simulink model "Basic_DMT"  (R2014b)
settings: Solver=FixedStepDiscrete  SolverMode=SingleTasking  StartTime=0.0  StopTime=25e-6-14e-9*24  RelTol=1e-3
PreLoadFcn:
  | userName = getenv('UserName');
  | 
  | if strcmp(userName,'Tim')
  | cd C:\Users\Tim\Documents\GitHub\MA_1\Basic_DMT
  | else
  | cd C:\Users\Tim-UML\Documents\GitHub\MA_1\Basic_DMT
  | end
InitFcn:
  | userName = getenv('UserName');
  | 
  | if strcmp(userName,'Tim')
  | cd C:\Users\Tim\Documents\GitHub\MA_1\Basic_DMT
  | else
  | cd C:\Users\Tim-UML\Documents\GitHub\MA_1\Basic_DMT
  | end
values from neighbouring files (symbols this model uses):
  a0 = 0.21194908595403703    (= 0.211949085954)    [initScript.m]
  a1 = 0.576101828091926    (= 0.576101828092)    [initScript.m]
  a2 = a0    (= 0.211949085954)    [initScript.m]
  beta = 1    [initScript.m]
  bitPerSymb = 4    [initScript.m]
  chanDownFact = Tchan/SystemPeriod    [initScript.m]
  fftLen = 16    [initScript.m]
  fftLenActive = fftLenDMT    (= 32)    [initScript.m]
  fftLenDMT = 2*fftLen    (= 32)    [initScript.m]
  GI_Active = GI_LenDMT    (= 0)    [initScript.m]
  GI_Len = 0    [initScript.m]
  GI_LenDMT = 0    [initScript.m]
  M = log2(fftLen)    [initScript.m]
  sysgenSystemPeriod = 4e-9    (= 4e-09)    [initScript.m]
  SystemPeriod = 4e-9    (= 4e-09)    [initScript.m]
  upsampleFactor = 1    [initScript.m]
  usedSubCar = 14    [initScript.m]
undefined symbols (not defined in the file or in its folder): bitCount, get, modu_mode, Tb, Ts
libraries: xbsIndex_r4 x822, commdigbbndam3 x59, simulink x42, dspsigops x7, commrandsrc2 x6, dspbuff3 x4, dspxfrm3 x3, dspswit3 x2, commseqgen2 x1, dsparch4 x1, commutil2 x1, dspsnks4 x1
(part 9 of 10)

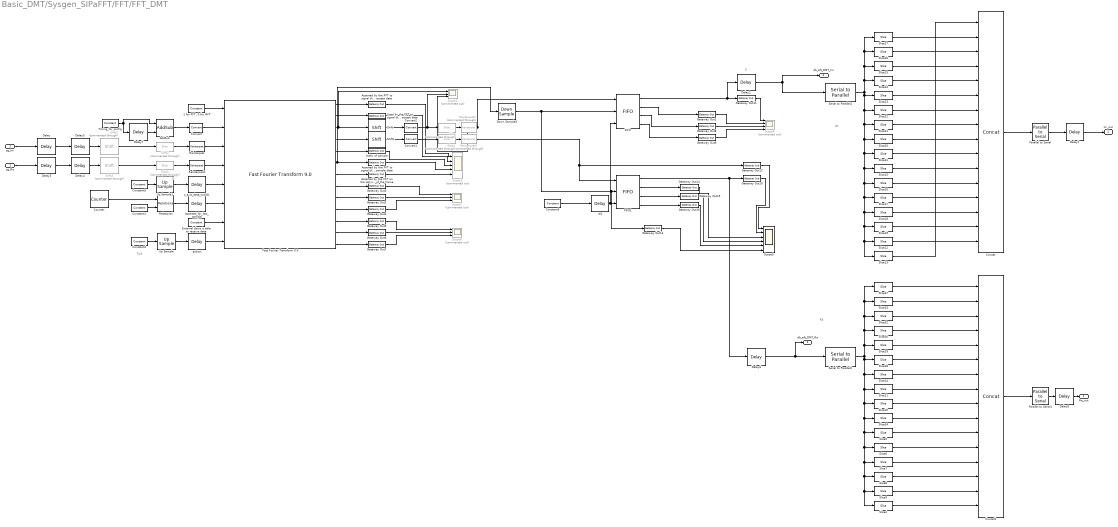
== system Basic_DMT/Sysgen_SIPaFFT/FFT/FFT_DMT ==
  note: 5
  note: IM
  note: RE
  note: 6
  note: Ts/3
  sg_Re : Inport
  sg_Im : Inport  Port=2
  "1 for FFT, 0 for IFFT " : xbsIndex_r4/Constant  const=1  gui_display_data_type=Fixed-point  arith_type=Unsigned  n_bits=1  bin_pt=0  preci_type=Single  exp_width=8  frac_width=24  explicit_period=on  period=Ts  equ=P=C  opselect=C  inp2=PCIN>>17  opr=+  inp1=P  carry=CIN  dbl_ovrd=off  block_type=constant
  AddSub : xbsIndex_r4/AddSub  mode=Subtraction  use_carryin=off  use_carryout=off  en=off  latency=0  precision=User Defined  arith_type=Unsigned  n_bits=1  bin_pt=0  quantization=Truncate  overflow=Wrap  use_behavioral_HDL=off  hw_selection=Fabric  pipelined=off  dbl_ovrd=off  block_type=addsub
  "Asserted by the FFT on the last sample of the frame " : xbsIndex_r4/Gateway Out  inherit_from_input=off  hdl_port=off  rows=1  columns=1  UseAsDAC=off  DACChannel='1'  interface=None  automatic_assignment=on  address_offset=hex2dec('00')  intf_description=''  timing_constraint=None  locs_specified=off  LOCs={}  io_standard={}  block_type=gatewayout
  "Asserted by the FFT to signal that it is ready to accept data " : xbsIndex_r4/Gateway Out  inherit_from_input=off  hdl_port=off  rows=1  columns=1  UseAsDAC=off  DACChannel='1'  interface=None  automatic_assignment=on  address_offset=hex2dec('00')  intf_description=''  timing_constraint=None  locs_specified=off  LOCs={}  io_standard={}  block_type=gatewayout
  Asserted by the FFT to signal that it is ready to provide sample data : xbsIndex_r4/Gateway Out  inherit_from_input=off  hdl_port=off  rows=1  columns=1  UseAsDAC=off  DACChannel='1'  interface=None  automatic_assignment=on  address_offset=hex2dec('00')  intf_description=''  timing_constraint=None  locs_specified=off  LOCs={}  io_standard={}  block_type=gatewayout
  Asserted_for_last_sample : xbsIndex_r4/Delay  rst=off  infoeditControl=Selection of Reset will increase slice count due to use of real FFs and instead of SRLs  en=off  latency=1  reg_retiming=off  dbl_ovrd=off  block_type=delay
  Concat : xbsIndex_r4/Concat  num_inputs=16  dbl_ovrd=off  block_type=concat
  Concat1 : xbsIndex_r4/Concat  num_inputs=16  dbl_ovrd=off  block_type=concat
  Constant1 : xbsIndex_r4/Constant  const=fftLenDMT-1  gui_display_data_type=Fixed-point  arith_type=Unsigned  n_bits=log2(fftLenDMT)  bin_pt=0  preci_type=Single  exp_width=8  frac_width=24  explicit_period=on  period=Ts*usedSubCar*bitPerSymb/fftLenDMT  equ=P=C  opselect=C  inp2=PCIN>>17  opr=+  inp1=P  carry=CIN  dbl_ovrd=off  block_type=constant
  Constant3 : xbsIndex_r4/Constant  const=1  gui_display_data_type=Boolean  arith_type=Boolean  n_bits=1  bin_pt=0  preci_type=Single  exp_width=8  frac_width=24  explicit_period=on  period=Ts*usedSubCar*bitPerSymb/fftLenDMT  equ=P=C  opselect=C  inp2=PCIN>>17  opr=+  inp1=P  carry=CIN  dbl_ovrd=off  block_type=constant
  Constant4 : xbsIndex_r4/Constant  const=1  gui_display_data_type=Boolean  arith_type=Boolean  n_bits=1  bin_pt=0  preci_type=Single  exp_width=8  frac_width=24  explicit_period=on  period=sysgenSystemPeriod*2  equ=P=C  opselect=C  inp2=PCIN>>17  opr=+  inp1=P  carry=CIN  dbl_ovrd=off  block_type=constant
  Constant5 : xbsIndex_r4/Constant  const=1  gui_display_data_type=Boolean  arith_type=Boolean  n_bits=1  bin_pt=0  preci_type=Single  exp_width=8  frac_width=24  explicit_period=on  period=Ts*usedSubCar*bitPerSymb/fftLenDMT  equ=P=C  opselect=C  inp2=PCIN>>17  opr=+  inp1=P  carry=CIN  dbl_ovrd=off  block_type=constant
  Convert : xbsIndex_r4/Convert  gui_display_data_type=Boolean  arith_type=Boolean  n_bits=1  bin_pt=0  float_type=Single  exp_bits=8  fraction_bits=24  quantization=Truncate  overflow=Wrap  en=off  latency=1  pipeline=off  dbl_ovrd=off  block_type=convert
  Convert1 : xbsIndex_r4/Convert  gui_display_data_type=Fixed-point  arith_type="Signed  (2's comp)"  n_bits=bitCount+(log2(fftLen)+1)*2  bin_pt=fracLen  float_type=Single  exp_bits=8  fraction_bits=24  quantization="Round  (unbiased: +/- Inf)"  overflow=Saturate  en=off  latency=0  pipeline=off  dbl_ovrd=off  block_type=convert
  Convert2 : xbsIndex_r4/Convert  gui_display_data_type=Fixed-point  arith_type="Signed  (2's comp)"  n_bits=bitCount+(log2(fftLen)+1)*2  bin_pt=fracLen  float_type=Single  exp_bits=8  fraction_bits=24  quantization="Round  (unbiased: +/- Inf)"  overflow=Saturate  en=off  latency=0  pipeline=off  dbl_ovrd=off  block_type=convert
  Counter : xbsIndex_r4/Counter  cnt_type=Count Limited  cnt_to=fftLenDMT-1  operation=Up  start_count=0  cnt_by_val=1  arith_type=Unsigned  n_bits=log2(fftLenDMT)  bin_pt=0  load_pin=off  rst=off  en=off  explicit_period=on  period=Ts*usedSubCar*bitPerSymb/fftLenDMT  use_behavioral_HDL=off  implementation=Fabric  dbl_ovrd=off  block_type=counter
  Delay : xbsIndex_r4/Delay  rst=off  infoeditControl=Selection of Reset will increase slice count due to use of real FFs and instead of SRLs  en=off  latency=1  reg_retiming=off  dbl_ovrd=off  block_type=delay
  Delay1 : xbsIndex_r4/Delay  rst=off  infoeditControl=Selection of Reset will increase slice count due to use of real FFs and instead of SRLs  en=off  latency=3  reg_retiming=off  dbl_ovrd=off  block_type=delay
  Delay2 : xbsIndex_r4/Delay  rst=off  infoeditControl=Selection of Reset will increase slice count due to use of real FFs and instead of SRLs  en=off  latency=6  reg_retiming=off  dbl_ovrd=off  block_type=delay
  Delay3 : xbsIndex_r4/Delay  rst=off  infoeditControl=Selection of Reset will increase slice count due to use of real FFs and instead of SRLs  en=off  latency=1  reg_retiming=off  dbl_ovrd=off  block_type=delay
  Delay4 : xbsIndex_r4/Delay  rst=off  infoeditControl=Selection of Reset will increase slice count due to use of real FFs and instead of SRLs  en=off  latency=16  reg_retiming=off  dbl_ovrd=off  block_type=delay
  Delay5 : xbsIndex_r4/Delay  rst=off  infoeditControl=Selection of Reset will increase slice count due to use of real FFs and instead of SRLs  en=off  latency=16  reg_retiming=off  dbl_ovrd=off  block_type=delay
  Delay6 : xbsIndex_r4/Delay  rst=off  infoeditControl=Selection of Reset will increase slice count due to use of real FFs and instead of SRLs  en=off  latency=6  reg_retiming=off  dbl_ovrd=off  block_type=delay
  Delay7 : xbsIndex_r4/Delay  rst=off  infoeditControl=Selection of Reset will increase slice count due to use of real FFs and instead of SRLs  en=off  latency=1  reg_retiming=off  dbl_ovrd=off  block_type=delay
  Delay8 : xbsIndex_r4/Delay  rst=off  infoeditControl=Selection of Reset will increase slice count due to use of real FFs and instead of SRLs  en=off  latency=3  reg_retiming=off  dbl_ovrd=off  block_type=delay
  Down Sample5 : xbsIndex_r4/Down Sample  sample_ratio=2  sample_phase=First Value of Frame  en=off  rst=off  latency=0  dbl_ovrd=off  block_type=dsamp
  "Externel slave is able to receive data " : xbsIndex_r4/Constant  const=1  gui_display_data_type=Boolean  arith_type=Boolean  n_bits=1  bin_pt=0  preci_type=Single  exp_width=8  frac_width=24  explicit_period=on  period=Ts  equ=P=C  opselect=C  inp2=PCIN>>17  opr=+  inp1=P  carry=CIN  dbl_ovrd=off  block_type=constant
  FIFO : xbsIndex_r4/FIFO  mem_type=Block RAM  performance_options=Standard_FIFO  embedded_registers=off  depth=32  percent_nbits=4  rst=off  rst_latency=1  en=off  use_dcount=off  use_percent_full_port=on  use_almost_empty=off  almost_empty_thresh=2  use_almost_full=off  almost_full_thresh=14  explicit_period=off  dbl_ovrd=off  block_type=fifo
  FIFO1 : xbsIndex_r4/FIFO  mem_type=Block RAM  performance_options=Standard_FIFO  embedded_registers=off  depth=32  percent_nbits=4  rst=off  rst_latency=1  en=off  use_dcount=off  use_percent_full_port=on  use_almost_empty=off  almost_empty_thresh=2  use_almost_full=off  almost_full_thresh=14  explicit_period=off  dbl_ovrd=off  block_type=fifo
  "Fast Fourier Transform 9.0 " : xbsIndex_r4/Fast Fourier Transform 9.0   transform_length=32  target_clock_frequency=250  target_data_throughput=50  implementation_options=pipelined_streaming_io  run_time_configurable_transform_length=off  phase_factor_width=20  scaling_options=unscaled  rounding_modes=convergent_rounding  aclken=on  aresetn=off  cyclic_prefix_insertion=off  output_ordering=natural_order  throttle_scheme=nonrealtime  xk_index=on  ovflo=off  trim_axipin_name=off  memory_options_data=block_ram  memory_options_phase_factors=block_ram  number_of_stages_using_block_ram_for_data_and_phase_factors=0  memory_options_reorder=block_ram  memory_options_hybrid=off  complex_mult_type=use_mults_resources  butterfly_type=use_xtremedsp_slices  channels=1  input_ordering=natural_order  input_width=16  ip_name=Fast Fourier Transform  ip_version=9.0  dsptool_ready=true  ipcore_usecache=true  ipcore_useipmodelcache=true  wrapper_available=true  port_translation_map={ 'aclken' => 'en', 'aresetn' => 'rst'}  data_format=fixed_point  block_type=xfft_v9_0
  Gateway Out{1..16} (16 alike) : xbsIndex_r4/Gateway Out  inherit_from_input=off  hdl_port=off  rows=1  columns=1  UseAsDAC=off  DACChannel='1'  interface=None  automatic_assignment=on  address_offset=hex2dec('00')  intf_description=''  timing_constraint=None  locs_specified=off  LOCs={}  io_standard={}  block_type=gatewayout
  Index of sample : xbsIndex_r4/Gateway Out  inherit_from_input=off  hdl_port=off  rows=1  columns=1  UseAsDAC=off  DACChannel='1'  interface=None  automatic_assignment=on  address_offset=hex2dec('00')  intf_description=''  timing_constraint=None  locs_specified=off  LOCs={}  io_standard={}  block_type=gatewayout
  Parallel to Serial : xbsIndex_r4/Parallel to Serial  output_order=Most Significant Word First  arith_type=Unsigned  output_bits=(bitCount+(log2(fftLen)+1)*2)  bin_pt=0  rst=off  en=off  latency=1  dbl_ovrd=off  block_type=p2s
      settings: infoedit=Each sample presented at the input becomes several samples presented serially at the output.
  Parallel to Serial1 : xbsIndex_r4/Parallel to Serial  output_order=Most Significant Word First  arith_type=Unsigned  output_bits=(bitCount+(log2(fftLen)+1)*2)  bin_pt=0  rst=off  en=off  latency=1  dbl_ovrd=off  block_type=p2s
      settings: infoedit=Each sample presented at the input becomes several samples presented serially at the output.
  Reinterpret : xbsIndex_r4/Reinterpret  force_arith_type=on  arith_type="Signed  (2's comp)"  force_bin_pt=on  bin_pt=bitCount-1+log2(fftLen)+1  block_type=reinterpret
  Reinterpret1 : xbsIndex_r4/Reinterpret  force_arith_type=on  arith_type="Signed  (2's comp)"  force_bin_pt=on  bin_pt=bitCount-1+log2(fftLen)+1  block_type=reinterpret
  Reinterpret2 : xbsIndex_r4/Reinterpret  Commented=through  force_arith_type=on  arith_type="Signed  (2's comp)"  force_bin_pt=on  bin_pt=fracLen  block_type=reinterpret
  Reinterpret3 : xbsIndex_r4/Reinterpret  Commented=through  force_arith_type=on  arith_type="Signed  (2's comp)"  force_bin_pt=on  bin_pt=fracLen  block_type=reinterpret
  Relational : xbsIndex_r4/Relational  mode=a=b  op_type=Bool  en=off  latency=0  dbl_ovrd=off  block_type=relational
  Scope1 : Scope  Commented=on  NumInputPorts=3
      settings: YMin=-5~-5~-5  YMax=5~5~5  SaveName=ScopeData42
  Scope2 : Scope  Commented=on  NumInputPorts=3
      settings: YMin=-5~-5~-5  YMax=5~5~5  SaveName=ScopeData49
  Scope3 : Scope  Commented=on  NumInputPorts=5
      settings: YMin=-5~-5~-5~-5~-5  YMax=5~5~5~5~5  SaveName=ScopeData51
  Scope4 : Scope  Commented=on  NumInputPorts=4
      settings: YMin=-5~-5~-5~-5  YMax=5~5~5~5  SaveName=ScopeData55
  Scope5 : Scope  NumInputPorts=6
      settings: YMin=-5~-5~-5~-5~-5~-5  YMax=5~5~5~5~5~5  SaveName=ScopeData56
  Scope8 : Scope  Commented=on  NumInputPorts=3
      settings: YMin=-5~-5~-5  YMax=5~5~5  SaveName=ScopeData57
  Serial to Parallel1 : xbsIndex_r4/Serial to Parallel  input_order=Most Significant Word First  arith_type=Unsigned  output_bits=(bitCount+(log2(fftLen)+1)*2)*fftLenDMT  bin_pt=0  rst=off  en=off  latency=1  dbl_ovrd=off  block_type=s2p
      settings: infoedit=Groups of samples presented serially at the input become single samples presented at the output.
  Serial to Parallel2 : xbsIndex_r4/Serial to Parallel  input_order=Most Significant Word First  arith_type=Unsigned  output_bits=(bitCount+(log2(fftLen)+1)*2)*fftLenDMT  bin_pt=0  rst=off  en=off  latency=1  dbl_ovrd=off  block_type=s2p
      settings: infoedit=Groups of samples presented serially at the input become single samples presented at the output.
  Shift : xbsIndex_r4/Shift  shift_dir=Left  shift_bits=2  en=off  latency=0  precision=Full  arith_type="Signed  (2's comp)"  n_bits=13  bin_pt=4  quantization="Round  (unbiased: +/- Inf)"  overflow=Saturate  dbl_ovrd=off  block_type=shift
  Shift1 : xbsIndex_r4/Shift  shift_dir=Left  shift_bits=2  en=off  latency=0  precision=Full  arith_type="Signed  (2's comp)"  n_bits=13  bin_pt=4  quantization="Round  (unbiased: +/- Inf)"  overflow=Saturate  dbl_ovrd=off  block_type=shift
  Shift2 : xbsIndex_r4/Shift  Commented=through  shift_dir=Right  shift_bits=1  en=off  latency=1  precision=Full  arith_type="Signed  (2's comp)"  n_bits=13  bin_pt=4  quantization="Round  (unbiased: +/- Inf)"  overflow=Saturate  dbl_ovrd=off  block_type=shift
  Shift3 : xbsIndex_r4/Shift  Commented=through  shift_dir=Right  shift_bits=1  en=off  latency=1  precision=Full  arith_type="Signed  (2's comp)"  n_bits=13  bin_pt=4  quantization="Round  (unbiased: +/- Inf)"  overflow=Saturate  dbl_ovrd=off  block_type=shift
  Slice : xbsIndex_r4/Slice  Commented=through  nbits=13  boolean_output=off  mode=Lower Bit Location + Width  bit1=0  base1=MSB of Input  bit0=0  base0=LSB of Input  dbl_ovrd=off  block_type=slice
  Slice1 : xbsIndex_r4/Slice  Commented=through  nbits=13  boolean_output=off  mode=Lower Bit Location + Width  bit1=0  base1=MSB of Input  bit0=0  base0=LSB of Input  dbl_ovrd=off  block_type=slice
  Slice10 : xbsIndex_r4/Slice  nbits=(bitCount+(log2(fftLen)+1)*2)  boolean_output=off  mode=Lower Bit Location + Width  bit1=0  base1=LSB of Input  bit0=(bitCount+(log2(fftLen)+1)*2)*23  base0=LSB of Input  dbl_ovrd=off  block_type=slice
  Slice11 : xbsIndex_r4/Slice  nbits=(bitCount+(log2(fftLen)+1)*2)  boolean_output=off  mode=Lower Bit Location + Width  bit1=0  base1=LSB of Input  bit0=(bitCount+(log2(fftLen)+1)*2)*24  base0=LSB of Input  dbl_ovrd=off  block_type=slice
  Slice12 : xbsIndex_r4/Slice  nbits=(bitCount+(log2(fftLen)+1)*2)  boolean_output=off  mode=Lower Bit Location + Width  bit1=0  base1=MSB of Input  bit0=(bitCount+(log2(fftLen)+1)*2)*16  base0=LSB of Input  dbl_ovrd=off  block_type=slice
  Slice13 : xbsIndex_r4/Slice  nbits=(bitCount+(log2(fftLen)+1)*2)  boolean_output=off  mode=Lower Bit Location + Width  bit1=0  base1=MSB of Input  bit0=(bitCount+(log2(fftLen)+1)*2)*15  base0=LSB of Input  dbl_ovrd=off  block_type=slice
  Slice14 : xbsIndex_r4/Slice  nbits=(bitCount+(log2(fftLen)+1)*2)  boolean_output=off  mode=Lower Bit Location + Width  bit1=0  base1=LSB of Input  bit0=(bitCount+(log2(fftLen)+1)*2)*25  base0=LSB of Input  dbl_ovrd=off  block_type=slice
  Slice15 : xbsIndex_r4/Slice  nbits=(bitCount+(log2(fftLen)+1)*2)  boolean_output=off  mode=Lower Bit Location + Width  bit1=24  base1=LSB of Input  bit0=(bitCount+(log2(fftLen)+1)*2)*21  base0=LSB of Input  dbl_ovrd=off  block_type=slice
  Slice16 : xbsIndex_r4/Slice  nbits=(bitCount+(log2(fftLen)+1)*2)  boolean_output=off  mode=Lower Bit Location + Width  bit1=0  base1=MSB of Input  bit0=(bitCount+(log2(fftLen)+1)*2)*20  base0=LSB of Input  dbl_ovrd=off  block_type=slice
  Slice17 : xbsIndex_r4/Slice  nbits=(bitCount+(log2(fftLen)+1)*2)  boolean_output=off  mode=Lower Bit Location + Width  bit1=0  base1=MSB of Input  bit0=(bitCount+(log2(fftLen)+1)*2)*19  base0=LSB of Input  dbl_ovrd=off  block_type=slice
  Slice18 : xbsIndex_r4/Slice  nbits=(bitCount+(log2(fftLen)+1)*2)  boolean_output=off  mode=Lower Bit Location + Width  bit1=0  base1=MSB of Input  bit0=(bitCount+(log2(fftLen)+1)*2)*18  base0=LSB of Input  dbl_ovrd=off  block_type=slice
  Slice19 : xbsIndex_r4/Slice  nbits=(bitCount+(log2(fftLen)+1)*2)  boolean_output=off  mode=Lower Bit Location + Width  bit1=0  base1=MSB of Input  bit0=(bitCount+(log2(fftLen)+1)*2)*17  base0=LSB of Input  dbl_ovrd=off  block_type=slice
  Slice2 : xbsIndex_r4/Slice  Commented=through  nbits=16  boolean_output=off  mode=Lower Bit Location + Width  bit1=0  base1=MSB of Input  bit0=0  base0=LSB of Input  dbl_ovrd=off  block_type=slice
  Slice20 : xbsIndex_r4/Slice  nbits=(bitCount+(log2(fftLen)+1)*2)  boolean_output=off  mode=Lower Bit Location + Width  bit1=0  base1=LSB of Input  bit0=(bitCount+(log2(fftLen)+1)*2)*23  base0=LSB of Input  dbl_ovrd=off  block_type=slice
  Slice21 : xbsIndex_r4/Slice  nbits=(bitCount+(log2(fftLen)+1)*2)  boolean_output=off  mode=Lower Bit Location + Width  bit1=0  base1=LSB of Input  bit0=(bitCount+(log2(fftLen)+1)*2)*24  base0=LSB of Input  dbl_ovrd=off  block_type=slice
  Slice22 : xbsIndex_r4/Slice  nbits=(bitCount+(log2(fftLen)+1)*2)  boolean_output=off  mode=Lower Bit Location + Width  bit1=0  base1=LSB of Input  bit0=(bitCount+(log2(fftLen)+1)*2)*25  base0=LSB of Input  dbl_ovrd=off  block_type=slice
  Slice23 : xbsIndex_r4/Slice  nbits=(bitCount+(log2(fftLen)+1)*2)  boolean_output=off  mode=Lower Bit Location + Width  bit1=0  base1=LSB of Input  bit0=(bitCount+(log2(fftLen)+1)*2)*26  base0=LSB of Input  dbl_ovrd=off  block_type=slice
  Slice24 : xbsIndex_r4/Slice  nbits=(bitCount+(log2(fftLen)+1)*2)  boolean_output=off  mode=Lower Bit Location + Width  bit1=0  base1=LSB of Input  bit0=(bitCount+(log2(fftLen)+1)*2)*27  base0=LSB of Input  dbl_ovrd=off  block_type=slice
  Slice25 : xbsIndex_r4/Slice  nbits=(bitCount+(log2(fftLen)+1)*2)  boolean_output=off  mode=Lower Bit Location + Width  bit1=0  base1=LSB of Input  bit0=(bitCount+(log2(fftLen)+1)*2)*28  base0=LSB of Input  dbl_ovrd=off  block_type=slice
  Slice26 : xbsIndex_r4/Slice  nbits=(bitCount+(log2(fftLen)+1)*2)  boolean_output=off  mode=Lower Bit Location + Width  bit1=0  base1=LSB of Input  bit0=(bitCount+(log2(fftLen)+1)*2)*29  base0=LSB of Input  dbl_ovrd=off  block_type=slice
  Slice27 : xbsIndex_r4/Slice  nbits=(bitCount+(log2(fftLen)+1)*2)  boolean_output=off  mode=Lower Bit Location + Width  bit1=0  base1=LSB of Input  bit0=(bitCount+(log2(fftLen)+1)*2)*30  base0=LSB of Input  dbl_ovrd=off  block_type=slice
  Slice28 : xbsIndex_r4/Slice  nbits=(bitCount+(log2(fftLen)+1)*2)  boolean_output=off  mode=Lower Bit Location + Width  bit1=0  base1=LSB of Input  bit0=(bitCount+(log2(fftLen)+1)*2)*26  base0=LSB of Input  dbl_ovrd=off  block_type=slice
  Slice29 : xbsIndex_r4/Slice  nbits=(bitCount+(log2(fftLen)+1)*2)  boolean_output=off  mode=Lower Bit Location + Width  bit1=0  base1=LSB of Input  bit0=(bitCount+(log2(fftLen)+1)*2)*27  base0=LSB of Input  dbl_ovrd=off  block_type=slice
  Slice3 : xbsIndex_r4/Slice  Commented=through  nbits=16  boolean_output=off  mode=Lower Bit Location + Width  bit1=0  base1=MSB of Input  bit0=0  base0=LSB of Input  dbl_ovrd=off  block_type=slice
  Slice30 : xbsIndex_r4/Slice  nbits=(bitCount+(log2(fftLen)+1)*2)  boolean_output=off  mode=Lower Bit Location + Width  bit1=0  base1=LSB of Input  bit0=(bitCount+(log2(fftLen)+1)*2)*28  base0=LSB of Input  dbl_ovrd=off  block_type=slice
  Slice31 : xbsIndex_r4/Slice  nbits=(bitCount+(log2(fftLen)+1)*2)  boolean_output=off  mode=Lower Bit Location + Width  bit1=0  base1=LSB of Input  bit0=(bitCount+(log2(fftLen)+1)*2)*22  base0=LSB of Input  dbl_ovrd=off  block_type=slice
  Slice32 : xbsIndex_r4/Slice  nbits=(bitCount+(log2(fftLen)+1)*2)  boolean_output=off  mode=Lower Bit Location + Width  bit1=0  base1=LSB of Input  bit0=(bitCount+(log2(fftLen)+1)*2)*29  base0=LSB of Input  dbl_ovrd=off  block_type=slice
  Slice33 : xbsIndex_r4/Slice  nbits=(bitCount+(log2(fftLen)+1)*2)  boolean_output=off  mode=Lower Bit Location + Width  bit1=0  base1=LSB of Input  bit0=(bitCount+(log2(fftLen)+1)*2)*30  base0=LSB of Input  dbl_ovrd=off  block_type=slice
  Slice34 : xbsIndex_r4/Slice  nbits=(bitCount+(log2(fftLen)+1)*2)  boolean_output=off  mode=Lower Bit Location + Width  bit1=0  base1=LSB of Input  bit0=(bitCount+(log2(fftLen)+1)*2)*22  base0=LSB of Input  dbl_ovrd=off  block_type=slice
  Slice37 : xbsIndex_r4/Slice  nbits=(bitCount+(log2(fftLen)+1)*2)  boolean_output=off  mode=Lower Bit Location + Width  bit1=0  base1=LSB of Input  bit0=(bitCount+(log2(fftLen)+1)*2)*31  base0=LSB of Input  dbl_ovrd=off  block_type=slice
  Slice4 : xbsIndex_r4/Slice  nbits=(bitCount+(log2(fftLen)+1)*2)  boolean_output=off  mode=Lower Bit Location + Width  bit1=0  base1=MSB of Input  bit0=(bitCount+(log2(fftLen)+1)*2)*16  base0=LSB of Input  dbl_ovrd=off  block_type=slice
  Slice5 : xbsIndex_r4/Slice  nbits=(bitCount+(log2(fftLen)+1)*2)  boolean_output=off  mode=Lower Bit Location + Width  bit1=24  base1=LSB of Input  bit0=(bitCount+(log2(fftLen)+1)*2)*21  base0=LSB of Input  dbl_ovrd=off  block_type=slice
  Slice6 : xbsIndex_r4/Slice  nbits=(bitCount+(log2(fftLen)+1)*2)  boolean_output=off  mode=Lower Bit Location + Width  bit1=0  base1=MSB of Input  bit0=(bitCount+(log2(fftLen)+1)*2)*20  base0=LSB of Input  dbl_ovrd=off  block_type=slice
  Slice7 : xbsIndex_r4/Slice  nbits=(bitCount+(log2(fftLen)+1)*2)  boolean_output=off  mode=Lower Bit Location + Width  bit1=0  base1=MSB of Input  bit0=(bitCount+(log2(fftLen)+1)*2)*19  base0=LSB of Input  dbl_ovrd=off  block_type=slice
  Slice8 : xbsIndex_r4/Slice  nbits=(bitCount+(log2(fftLen)+1)*2)  boolean_output=off  mode=Lower Bit Location + Width  bit1=0  base1=MSB of Input  bit0=(bitCount+(log2(fftLen)+1)*2)*18  base0=LSB of Input  dbl_ovrd=off  block_type=slice
  Slice9 : xbsIndex_r4/Slice  nbits=(bitCount+(log2(fftLen)+1)*2)  boolean_output=off  mode=Lower Bit Location + Width  bit1=0  base1=MSB of Input  bit0=(bitCount+(log2(fftLen)+1)*2)*17  base0=LSB of Input  dbl_ovrd=off  block_type=slice
  Timing_for_config : xbsIndex_r4/Constant  const=1  gui_display_data_type=Fixed-point  arith_type=Unsigned  n_bits=1  bin_pt=0  preci_type=Single  exp_width=8  frac_width=24  explicit_period=on  period=Ts  equ=P=C  opselect=C  inp2=PCIN>>17  opr=+  inp1=P  carry=CIN  dbl_ovrd=off  block_type=constant
  Up Sample : xbsIndex_r4/Up Sample  sample_ratio=2  copy_samples=off  en=off  latency=0  dbl_ovrd=off  block_type=usamp
  Up Sample1 : xbsIndex_r4/Up Sample  sample_ratio=Ts*usedSubCar*bitPerSymb/fftLenDMT/sysgenSystemPeriod  copy_samples=off  en=off  latency=0  dbl_ovrd=off  block_type=usamp
  Used by the FFT to signal that it is ready to accept data : xbsIndex_r4/Gateway Out  inherit_from_input=off  hdl_port=off  rows=1  columns=1  UseAsDAC=off  DACChannel='1'  interface=None  automatic_assignment=on  address_offset=hex2dec('00')  intf_description=''  timing_constraint=None  locs_specified=off  LOCs={}  io_standard={}  block_type=gatewayout
  "aclken " : xbsIndex_r4/Delay  rst=off  infoeditControl=Selection of Reset will increase slice count due to use of real FFs and instead of SRLs  en=off  latency=1  reg_retiming=off  dbl_ovrd=off  block_type=delay
  re2 : xbsIndex_r4/Delay  rst=off  infoeditControl=Selection of Reset will increase slice count due to use of real FFs and instead of SRLs  en=off  latency=1  reg_retiming=off  dbl_ovrd=off  block_type=delay
  s_axis_data_tvalid1 : xbsIndex_r4/Delay  rst=off  infoeditControl=Selection of Reset will increase slice count due to use of real FFs and instead of SRLs  en=off  latency=1  reg_retiming=off  dbl_ovrd=off  block_type=delay
  Re_out : Outport
  Im_out : Outport  Port=2
  db_aft_DMT_Re : Outport  Port=3
  db_aft_DMT_Im : Outport  Port=4
  wires:
  "1 for FFT, 0 for IFFT "/1 -> "Fast Fourier Transform 9.0 "/1
  "Externel slave is able to receive data "/1 -> "Fast Fourier Transform 9.0 "/7
  "Fast Fourier Transform 9.0 "/4 -> Shift1/1
  Shift1/1 -> Convert1/1
  Slice/1 -> Reinterpret2/1
  Slice1/1 -> Reinterpret3/1
  Slice2/1 -> Reinterpret/1
  Slice3/1 -> Reinterpret1/1
  Shift/1 -> Convert2/1
  Delay/1 -> Delay5/1
  Delay3/1 -> Delay4/1
  Reinterpret2/1 -> FIFO/1, Scope1/3
  Reinterpret1/1 -> "Fast Fourier Transform 9.0 "/4
  Reinterpret/1 -> "Fast Fourier Transform 9.0 "/3
  Shift2/1 -> Slice2/1
  Shift3/1 -> Slice3/1
  Convert2/1 -> Slice/1, Scope1/2
  Convert1/1 -> Slice1/1
  "Fast Fourier Transform 9.0 "/6 -> Asserted by the FFT to signal that it is ready to provide sample data/1, Down Sample5/1
  "Fast Fourier Transform 9.0 "/7 -> "Asserted by the FFT on the last sample of the frame "/1
  "Fast Fourier Transform 9.0 "/10 -> Gateway Out4/1
  "Fast Fourier Transform 9.0 "/11 -> Gateway Out5/1
  "Fast Fourier Transform 9.0 "/12 -> Gateway Out6/1
  "Fast Fourier Transform 9.0 "/13 -> Gateway Out7/1
  "Fast Fourier Transform 9.0 "/9 -> Gateway Out2/1
  "Fast Fourier Transform 9.0 "/8 -> Gateway Out3/1
  Gateway Out6/1 -> Scope8/2
  Gateway Out7/1 -> Scope8/3
  Gateway Out5/1 -> Scope8/1
  Gateway Out2/1 -> Scope2/2
  Gateway Out3/1 -> Scope2/1
  Gateway Out4/1 -> Scope2/3
  Asserted by the FFT to signal that it is ready to provide sample data/1 -> Scope3/4
  "Asserted by the FFT on the last sample of the frame "/1 -> Scope3/5
  Index of sample/1 -> Scope3/3
  Used by the FFT to signal that it is ready to accept data/1 -> Scope3/2
  "Fast Fourier Transform 9.0 "/5 -> Index of sample/1
  "Fast Fourier Transform 9.0 "/1 -> "Asserted by the FFT to signal that it is ready to accept data "/1
  "Fast Fourier Transform 9.0 "/2 -> Used by the FFT to signal that it is ready to accept data/1
  "Asserted by the FFT to signal that it is ready to accept data "/1 -> Scope3/1
  AddSub/1 -> Convert/1
  Timing_for_config/1 -> Delay7/1, AddSub/1
  Delay7/1 -> AddSub/2
  Convert/1 -> "Fast Fourier Transform 9.0 "/2
  s_axis_data_tvalid1/1 -> "Fast Fourier Transform 9.0 "/5
  Relational/1 -> Asserted_for_last_sample/1
  Constant1/1 -> Relational/2
  Asserted_for_last_sample/1 -> "Fast Fourier Transform 9.0 "/6
  Counter/1 -> Relational/1
  Up Sample/1 -> "aclken "/1
  Constant4/1 -> Up Sample/1
  "aclken "/1 -> "Fast Fourier Transform 9.0 "/8
  Up Sample1/1 -> s_axis_data_tvalid1/1
  Constant5/1 -> Up Sample1/1
  Gateway Out8/1 -> Scope4/3
  Gateway Out9/1 -> Scope4/4
  Gateway Out1/1 -> Scope4/2
  FIFO/2 -> Gateway Out1/1
  FIFO/3 -> Gateway Out8/1
  FIFO/4 -> Gateway Out9/1
  Gateway Out15/1 -> Scope5/4
  Gateway Out16/1 -> Scope5/5
  Gateway Out14/1 -> Scope5/3
  FIFO1/2 -> Gateway Out14/1
  FIFO1/3 -> Gateway Out15/1
  FIFO1/4 -> Gateway Out16/1
  Gateway Out10/1 -> Scope5/2
  Gateway Out11/1 -> Scope4/1
  Gateway Out12/1 -> Scope5/1
  re2/1 -> FIFO/3, FIFO1/3
  Gateway Out13/1 -> Scope5/6
  FIFO/1 -> Delay2/1, Gateway Out11/1
  Reinterpret3/1 -> FIFO1/1, Gateway Out12/1
  Down Sample5/1 -> Gateway Out13/1, FIFO1/2, FIFO/2
  Constant3/1 -> re2/1
  sg_Im/1 -> Delay/1
  sg_Re/1 -> Delay3/1
  Slice27/1 -> Concat/2
  Slice26/1 -> Concat/3
  Slice25/1 -> Concat/4
  Slice24/1 -> Concat/5
  Slice23/1 -> Concat/6
  Slice22/1 -> Concat/7
  Slice21/1 -> Concat/8
  Slice20/1 -> Concat/9
  Slice15/1 -> Concat/11
  Slice16/1 -> Concat/12
  Slice17/1 -> Concat/13
  Slice18/1 -> Concat/14
  Slice31/1 -> Concat/10
  Concat/1 -> Parallel to Serial/1
  Slice12/1 -> Concat/16
  Slice19/1 -> Concat/15
  Slice33/1 -> Concat1/2
  Slice32/1 -> Concat1/3
  Slice30/1 -> Concat1/4
  Slice29/1 -> Concat1/5
  Slice28/1 -> Concat1/6
  Slice14/1 -> Concat1/7
  Slice11/1 -> Concat1/8
  Slice10/1 -> Concat1/9
  Slice5/1 -> Concat1/11
  Slice6/1 -> Concat1/12
  Slice7/1 -> Concat1/13
  Slice8/1 -> Concat1/14
  Serial to Parallel2/1 -> Slice28/1, Slice14/1, Slice11/1, Slice10/1, Slice34/1, Slice5/1, Slice6/1, Slice7/1, Slice8/1, Slice9/1, Slice4/1, Slice29/1, Slice30/1, Slice32/1, Slice33/1, Slice37/1
  Slice34/1 -> Concat1/10
  Concat1/1 -> Parallel to Serial1/1
  Slice4/1 -> Concat1/16
  Slice9/1 -> Concat1/15
  Slice13/1 -> Concat/1
  Slice37/1 -> Concat1/1
  Parallel to Serial1/1 -> Delay8/1
  Parallel to Serial/1 -> Delay1/1
  Serial to Parallel1/1 -> Slice15/1, Slice13/1, Slice12/1, Slice19/1, Slice18/1, Slice17/1, Slice16/1, Slice31/1, Slice20/1, Slice21/1, Slice22/1, Slice23/1, Slice26/1, Slice27/1, Slice25/1, Slice24/1
  Delay4/1 -> Shift3/1
  Delay5/1 -> Shift2/1
  "Fast Fourier Transform 9.0 "/3 -> Shift/1, Scope1/1
  FIFO1/1 -> Delay6/1, Gateway Out10/1
  Delay2/1 -> Serial to Parallel1/1, db_aft_DMT_Im/1
  Delay6/1 -> db_aft_DMT_Re/1, Serial to Parallel2/1
  Delay1/1 -> Im_out/1
  Delay8/1 -> Re_out/1

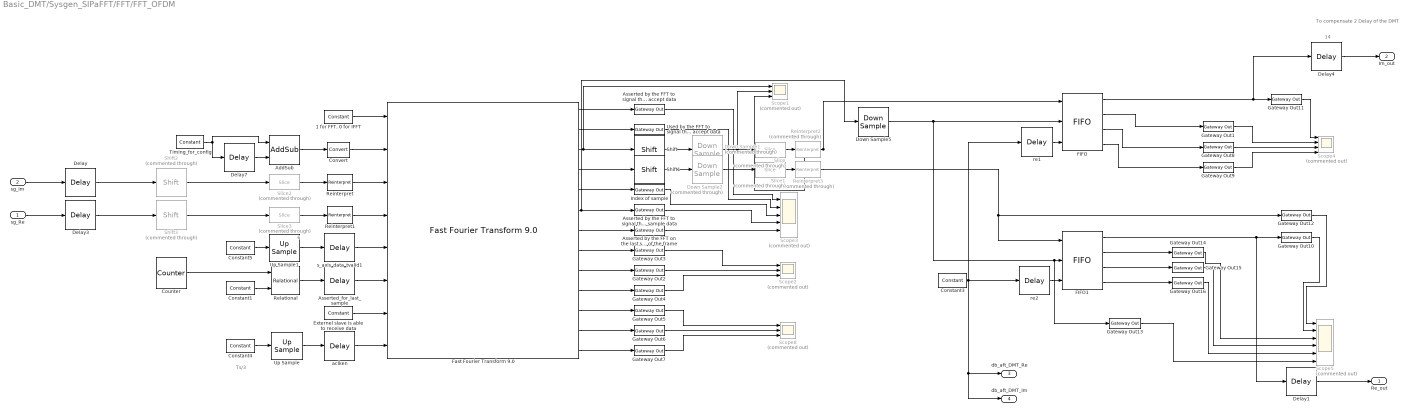
== system Basic_DMT/Sysgen_SIPaFFT/FFT/FFT_OFDM ==
  note: 14
  note: To compensate 2 Delay of the DMT
  note: 6
  note: Ts/3
  sg_Re : Inport
  sg_Im : Inport  Port=2
  "1 for FFT, 0 for IFFT " : xbsIndex_r4/Constant  const=1  gui_display_data_type=Fixed-point  arith_type=Unsigned  n_bits=1  bin_pt=0  preci_type=Single  exp_width=8  frac_width=24  explicit_period=on  period=Ts  equ=P=C  opselect=C  inp2=PCIN>>17  opr=+  inp1=P  carry=CIN  dbl_ovrd=off  block_type=constant
  AddSub : xbsIndex_r4/AddSub  mode=Subtraction  use_carryin=off  use_carryout=off  en=off  latency=0  precision=User Defined  arith_type=Unsigned  n_bits=1  bin_pt=0  quantization=Truncate  overflow=Wrap  use_behavioral_HDL=off  hw_selection=Fabric  pipelined=off  dbl_ovrd=off  block_type=addsub
  "Asserted by the FFT on the last sample of the frame " : xbsIndex_r4/Gateway Out  inherit_from_input=off  hdl_port=off  rows=1  columns=1  UseAsDAC=off  DACChannel='1'  interface=None  automatic_assignment=on  address_offset=hex2dec('00')  intf_description=''  timing_constraint=None  locs_specified=off  LOCs={}  io_standard={}  block_type=gatewayout
  "Asserted by the FFT to signal that it is ready to accept data " : xbsIndex_r4/Gateway Out  inherit_from_input=off  hdl_port=off  rows=1  columns=1  UseAsDAC=off  DACChannel='1'  interface=None  automatic_assignment=on  address_offset=hex2dec('00')  intf_description=''  timing_constraint=None  locs_specified=off  LOCs={}  io_standard={}  block_type=gatewayout
  Asserted by the FFT to signal that it is ready to provide sample data : xbsIndex_r4/Gateway Out  inherit_from_input=off  hdl_port=off  rows=1  columns=1  UseAsDAC=off  DACChannel='1'  interface=None  automatic_assignment=on  address_offset=hex2dec('00')  intf_description=''  timing_constraint=None  locs_specified=off  LOCs={}  io_standard={}  block_type=gatewayout
  Asserted_for_last_sample : xbsIndex_r4/Delay  rst=off  infoeditControl=Selection of Reset will increase slice count due to use of real FFs and instead of SRLs  en=off  latency=1  reg_retiming=off  dbl_ovrd=off  block_type=delay
  Constant1 : xbsIndex_r4/Constant  const=fftLen-1  gui_display_data_type=Fixed-point  arith_type=Unsigned  n_bits=log2(fftLen)  bin_pt=0  preci_type=Single  exp_width=8  frac_width=24  explicit_period=on  period=Ts*usedSubCar*bitPerSymb/fftLen  equ=P=C  opselect=C  inp2=PCIN>>17  opr=+  inp1=P  carry=CIN  dbl_ovrd=off  block_type=constant
  Constant3 : xbsIndex_r4/Constant  const=1  gui_display_data_type=Boolean  arith_type=Boolean  n_bits=1  bin_pt=0  preci_type=Single  exp_width=8  frac_width=24  explicit_period=on  period=Ts*usedSubCar*bitPerSymb/fftLen  equ=P=C  opselect=C  inp2=PCIN>>17  opr=+  inp1=P  carry=CIN  dbl_ovrd=off  block_type=constant
  Constant4 : xbsIndex_r4/Constant  const=1  gui_display_data_type=Boolean  arith_type=Boolean  n_bits=1  bin_pt=0  preci_type=Single  exp_width=8  frac_width=24  explicit_period=on  period=sysgenSystemPeriod*2  equ=P=C  opselect=C  inp2=PCIN>>17  opr=+  inp1=P  carry=CIN  dbl_ovrd=off  block_type=constant
  Constant5 : xbsIndex_r4/Constant  const=1  gui_display_data_type=Boolean  arith_type=Boolean  n_bits=1  bin_pt=0  preci_type=Single  exp_width=8  frac_width=24  explicit_period=on  period=Ts*usedSubCar*bitPerSymb/fftLen  equ=P=C  opselect=C  inp2=PCIN>>17  opr=+  inp1=P  carry=CIN  dbl_ovrd=off  block_type=constant
  Convert : xbsIndex_r4/Convert  gui_display_data_type=Boolean  arith_type=Boolean  n_bits=1  bin_pt=0  float_type=Single  exp_bits=8  fraction_bits=24  quantization=Truncate  overflow=Wrap  en=off  latency=1  pipeline=off  dbl_ovrd=off  block_type=convert
  Counter : xbsIndex_r4/Counter  cnt_type=Count Limited  cnt_to=fftLen-1  operation=Up  start_count=0  cnt_by_val=1  arith_type=Unsigned  n_bits=log2(fftLen)  bin_pt=0  load_pin=off  rst=off  en=off  explicit_period=on  period=Ts*usedSubCar*bitPerSymb/fftLen  use_behavioral_HDL=off  implementation=Fabric  dbl_ovrd=off  block_type=counter
  Delay : xbsIndex_r4/Delay  rst=off  infoeditControl=Selection of Reset will increase slice count due to use of real FFs and instead of SRLs  en=off  latency=1  reg_retiming=off  dbl_ovrd=off  block_type=delay
  Delay1 : xbsIndex_r4/Delay  rst=off  infoeditControl=Selection of Reset will increase slice count due to use of real FFs and instead of SRLs  en=off  latency=15  reg_retiming=off  dbl_ovrd=off  block_type=delay
  Delay3 : xbsIndex_r4/Delay  rst=off  infoeditControl=Selection of Reset will increase slice count due to use of real FFs and instead of SRLs  en=off  latency=1  reg_retiming=off  dbl_ovrd=off  block_type=delay
  Delay4 : xbsIndex_r4/Delay  rst=off  infoeditControl=Selection of Reset will increase slice count due to use of real FFs and instead of SRLs  en=off  latency=15  reg_retiming=off  dbl_ovrd=off  block_type=delay
  Delay7 : xbsIndex_r4/Delay  rst=off  infoeditControl=Selection of Reset will increase slice count due to use of real FFs and instead of SRLs  en=off  latency=1  reg_retiming=off  dbl_ovrd=off  block_type=delay
  Down Sample1 : xbsIndex_r4/Down Sample  Commented=through  sample_ratio=2  sample_phase="Last Value of Frame  (most efficient)"  en=off  rst=off  latency=1  dbl_ovrd=off  block_type=dsamp
  Down Sample2 : xbsIndex_r4/Down Sample  Commented=through  sample_ratio=2  sample_phase="Last Value of Frame  (most efficient)"  en=off  rst=off  latency=1  dbl_ovrd=off  block_type=dsamp
  Down Sample5 : xbsIndex_r4/Down Sample  sample_ratio=2  sample_phase=First Value of Frame  en=off  rst=off  latency=0  dbl_ovrd=off  block_type=dsamp
  "Externel slave is able to receive data " : xbsIndex_r4/Constant  const=1  gui_display_data_type=Boolean  arith_type=Boolean  n_bits=1  bin_pt=0  preci_type=Single  exp_width=8  frac_width=24  explicit_period=on  period=Ts  equ=P=C  opselect=C  inp2=PCIN>>17  opr=+  inp1=P  carry=CIN  dbl_ovrd=off  block_type=constant
  FIFO : xbsIndex_r4/FIFO  mem_type=Block RAM  performance_options=Standard_FIFO  embedded_registers=off  depth=16  percent_nbits=4  rst=off  rst_latency=1  en=off  use_dcount=off  use_percent_full_port=on  use_almost_empty=off  almost_empty_thresh=2  use_almost_full=off  almost_full_thresh=14  explicit_period=off  dbl_ovrd=off  block_type=fifo
  FIFO1 : xbsIndex_r4/FIFO  mem_type=Block RAM  performance_options=Standard_FIFO  embedded_registers=off  depth=16  percent_nbits=4  rst=off  rst_latency=1  en=off  use_dcount=off  use_percent_full_port=on  use_almost_empty=off  almost_empty_thresh=2  use_almost_full=off  almost_full_thresh=14  explicit_period=off  dbl_ovrd=off  block_type=fifo
  "Fast Fourier Transform 9.0 " : xbsIndex_r4/Fast Fourier Transform 9.0   transform_length=16  target_clock_frequency=250  target_data_throughput=50  implementation_options=pipelined_streaming_io  run_time_configurable_transform_length=off  phase_factor_width=20  scaling_options=unscaled  rounding_modes=convergent_rounding  aclken=on  aresetn=off  cyclic_prefix_insertion=off  output_ordering=natural_order  throttle_scheme=nonrealtime  xk_index=on  ovflo=off  trim_axipin_name=off  memory_options_data=block_ram  memory_options_phase_factors=block_ram  number_of_stages_using_block_ram_for_data_and_phase_factors=0  memory_options_reorder=block_ram  memory_options_hybrid=off  complex_mult_type=use_mults_resources  butterfly_type=use_xtremedsp_slices  channels=1  input_ordering=natural_order  input_width=16  ip_name=Fast Fourier Transform  ip_version=9.0  dsptool_ready=true  ipcore_usecache=true  ipcore_useipmodelcache=true  wrapper_available=true  port_translation_map={ 'aclken' => 'en', 'aresetn' => 'rst'}  data_format=fixed_point  block_type=xfft_v9_0
  Gateway Out{1..16} (16 alike) : xbsIndex_r4/Gateway Out  inherit_from_input=off  hdl_port=off  rows=1  columns=1  UseAsDAC=off  DACChannel='1'  interface=None  automatic_assignment=on  address_offset=hex2dec('00')  intf_description=''  timing_constraint=None  locs_specified=off  LOCs={}  io_standard={}  block_type=gatewayout
  Index of sample : xbsIndex_r4/Gateway Out  inherit_from_input=off  hdl_port=off  rows=1  columns=1  UseAsDAC=off  DACChannel='1'  interface=None  automatic_assignment=on  address_offset=hex2dec('00')  intf_description=''  timing_constraint=None  locs_specified=off  LOCs={}  io_standard={}  block_type=gatewayout
  Reinterpret : xbsIndex_r4/Reinterpret  force_arith_type=on  arith_type="Signed  (2's comp)"  force_bin_pt=on  bin_pt=bitCount-1+log2(fftLen)+1  block_type=reinterpret
  Reinterpret1 : xbsIndex_r4/Reinterpret  force_arith_type=on  arith_type="Signed  (2's comp)"  force_bin_pt=on  bin_pt=bitCount-1+log2(fftLen)+1  block_type=reinterpret
  Reinterpret2 : xbsIndex_r4/Reinterpret  Commented=through  force_arith_type=on  arith_type="Signed  (2's comp)"  force_bin_pt=on  bin_pt=fracLen  block_type=reinterpret
  Reinterpret3 : xbsIndex_r4/Reinterpret  Commented=through  force_arith_type=on  arith_type="Signed  (2's comp)"  force_bin_pt=on  bin_pt=fracLen  block_type=reinterpret
  Relational : xbsIndex_r4/Relational  mode=a=b  op_type=Bool  en=off  latency=0  dbl_ovrd=off  block_type=relational
  Scope1 : Scope  Commented=on  NumInputPorts=3
      settings: YMin=-5~-5~-5  YMax=5~5~5
  Scope2 : Scope  Commented=on  NumInputPorts=3
      settings: YMin=-5~-5~-5  YMax=5~5~5  SaveName=ScopeData35
  Scope3 : Scope  Commented=on  NumInputPorts=5
      settings: YMin=-5~-5~-5~-5~-5  YMax=5~5~5~5~5  SaveName=ScopeData36
  Scope4 : Scope  Commented=on  NumInputPorts=4
      settings: YMin=-5~-5~-5~-5  YMax=5~5~5~5  SaveName=ScopeData39
  Scope5 : Scope  Commented=on  NumInputPorts=6
      settings: YMin=-5~-5~-5~-5~-5~-5  YMax=5~5~5~5~5~5  SaveName=ScopeData43
  Scope8 : Scope  Commented=on  NumInputPorts=3
      settings: YMin=-5~-5~-5  YMax=5~5~5  SaveName=ScopeData37
  Shift : xbsIndex_r4/Shift  shift_dir=Right  shift_bits=log2(fftLen)  en=off  latency=0  precision=Full  arith_type="Signed  (2's comp)"  n_bits=13  bin_pt=4  quantization="Round  (unbiased: +/- Inf)"  overflow=Saturate  dbl_ovrd=off  block_type=shift
  Shift1 : xbsIndex_r4/Shift  shift_dir=Right  shift_bits=log2(fftLen)  en=off  latency=0  precision=Full  arith_type="Signed  (2's comp)"  n_bits=13  bin_pt=4  quantization="Round  (unbiased: +/- Inf)"  overflow=Saturate  dbl_ovrd=off  block_type=shift
  Shift2 : xbsIndex_r4/Shift  Commented=through  shift_dir=Right  shift_bits=1  en=off  latency=1  precision=Full  arith_type="Signed  (2's comp)"  n_bits=13  bin_pt=4  quantization="Round  (unbiased: +/- Inf)"  overflow=Saturate  dbl_ovrd=off  block_type=shift
  Shift3 : xbsIndex_r4/Shift  Commented=through  shift_dir=Right  shift_bits=1  en=off  latency=1  precision=Full  arith_type="Signed  (2's comp)"  n_bits=13  bin_pt=4  quantization="Round  (unbiased: +/- Inf)"  overflow=Saturate  dbl_ovrd=off  block_type=shift
  Slice : xbsIndex_r4/Slice  Commented=through  nbits=13  boolean_output=off  mode=Lower Bit Location + Width  bit1=0  base1=MSB of Input  bit0=0  base0=LSB of Input  dbl_ovrd=off  block_type=slice
  Slice1 : xbsIndex_r4/Slice  Commented=through  nbits=13  boolean_output=off  mode=Lower Bit Location + Width  bit1=0  base1=MSB of Input  bit0=0  base0=LSB of Input  dbl_ovrd=off  block_type=slice
  Slice2 : xbsIndex_r4/Slice  Commented=through  nbits=16  boolean_output=off  mode=Lower Bit Location + Width  bit1=0  base1=MSB of Input  bit0=0  base0=LSB of Input  dbl_ovrd=off  block_type=slice
  Slice3 : xbsIndex_r4/Slice  Commented=through  nbits=16  boolean_output=off  mode=Lower Bit Location + Width  bit1=0  base1=MSB of Input  bit0=0  base0=LSB of Input  dbl_ovrd=off  block_type=slice
  Timing_for_config : xbsIndex_r4/Constant  const=1  gui_display_data_type=Fixed-point  arith_type=Unsigned  n_bits=1  bin_pt=0  preci_type=Single  exp_width=8  frac_width=24  explicit_period=on  period=Ts  equ=P=C  opselect=C  inp2=PCIN>>17  opr=+  inp1=P  carry=CIN  dbl_ovrd=off  block_type=constant
  Up Sample : xbsIndex_r4/Up Sample  sample_ratio=2  copy_samples=off  en=off  latency=0  dbl_ovrd=off  block_type=usamp
  Up Sample1 : xbsIndex_r4/Up Sample  sample_ratio=Ts*usedSubCar*bitPerSymb/fftLen/sysgenSystemPeriod  copy_samples=off  en=off  latency=0  dbl_ovrd=off  block_type=usamp
  Used by the FFT to signal that it is ready to accept data : xbsIndex_r4/Gateway Out  inherit_from_input=off  hdl_port=off  rows=1  columns=1  UseAsDAC=off  DACChannel='1'  interface=None  automatic_assignment=on  address_offset=hex2dec('00')  intf_description=''  timing_constraint=None  locs_specified=off  LOCs={}  io_standard={}  block_type=gatewayout
  "aclken " : xbsIndex_r4/Delay  rst=off  infoeditControl=Selection of Reset will increase slice count due to use of real FFs and instead of SRLs  en=off  latency=1  reg_retiming=off  dbl_ovrd=off  block_type=delay
  re1 : xbsIndex_r4/Delay  rst=off  infoeditControl=Selection of Reset will increase slice count due to use of real FFs and instead of SRLs  en=off  latency=1  reg_retiming=off  dbl_ovrd=off  block_type=delay
  re2 : xbsIndex_r4/Delay  rst=off  infoeditControl=Selection of Reset will increase slice count due to use of real FFs and instead of SRLs  en=off  latency=1  reg_retiming=off  dbl_ovrd=off  block_type=delay
  s_axis_data_tvalid1 : xbsIndex_r4/Delay  rst=off  infoeditControl=Selection of Reset will increase slice count due to use of real FFs and instead of SRLs  en=off  latency=1  reg_retiming=off  dbl_ovrd=off  block_type=delay
  Re_out : Outport
  Im_out : Outport  Port=2
  db_aft_DMT_Re : Outport  Port=3
  db_aft_DMT_Im : Outport  Port=4
  wires:
  "1 for FFT, 0 for IFFT "/1 -> "Fast Fourier Transform 9.0 "/1
  "Externel slave is able to receive data "/1 -> "Fast Fourier Transform 9.0 "/7
  "Fast Fourier Transform 9.0 "/4 -> Shift1/1
  Shift1/1 -> Down Sample2/1
  Slice/1 -> Reinterpret2/1
  Slice1/1 -> Reinterpret3/1
  Slice2/1 -> Reinterpret/1
  Slice3/1 -> Reinterpret1/1
  "Fast Fourier Transform 9.0 "/3 -> Shift/1, Scope1/1
  Shift/1 -> Down Sample1/1
  Delay/1 -> Shift2/1
  Delay3/1 -> Shift3/1
  Reinterpret2/1 -> FIFO/1, Scope1/3
  Reinterpret1/1 -> "Fast Fourier Transform 9.0 "/4
  Reinterpret/1 -> "Fast Fourier Transform 9.0 "/3
  Shift2/1 -> Slice2/1
  Shift3/1 -> Slice3/1
  Down Sample1/1 -> Slice/1, Scope1/2
  Down Sample2/1 -> Slice1/1
  "Fast Fourier Transform 9.0 "/6 -> Asserted by the FFT to signal that it is ready to provide sample data/1, Down Sample5/1
  "Fast Fourier Transform 9.0 "/7 -> "Asserted by the FFT on the last sample of the frame "/1
  "Fast Fourier Transform 9.0 "/10 -> Gateway Out4/1
  "Fast Fourier Transform 9.0 "/11 -> Gateway Out5/1
  "Fast Fourier Transform 9.0 "/12 -> Gateway Out6/1
  "Fast Fourier Transform 9.0 "/13 -> Gateway Out7/1
  "Fast Fourier Transform 9.0 "/9 -> Gateway Out2/1
  "Fast Fourier Transform 9.0 "/8 -> Gateway Out3/1
  Gateway Out6/1 -> Scope8/2
  Gateway Out7/1 -> Scope8/3
  Gateway Out5/1 -> Scope8/1
  Gateway Out2/1 -> Scope2/2
  Gateway Out3/1 -> Scope2/1
  Gateway Out4/1 -> Scope2/3
  Asserted by the FFT to signal that it is ready to provide sample data/1 -> Scope3/4
  "Asserted by the FFT on the last sample of the frame "/1 -> Scope3/5
  Index of sample/1 -> Scope3/3
  Used by the FFT to signal that it is ready to accept data/1 -> Scope3/2
  "Fast Fourier Transform 9.0 "/5 -> Index of sample/1
  "Fast Fourier Transform 9.0 "/1 -> "Asserted by the FFT to signal that it is ready to accept data "/1
  "Fast Fourier Transform 9.0 "/2 -> Used by the FFT to signal that it is ready to accept data/1
  "Asserted by the FFT to signal that it is ready to accept data "/1 -> Scope3/1
  AddSub/1 -> Convert/1
  Timing_for_config/1 -> Delay7/1, AddSub/1
  Delay7/1 -> AddSub/2
  Convert/1 -> "Fast Fourier Transform 9.0 "/2
  s_axis_data_tvalid1/1 -> "Fast Fourier Transform 9.0 "/5
  Relational/1 -> Asserted_for_last_sample/1
  Constant1/1 -> Relational/2
  Asserted_for_last_sample/1 -> "Fast Fourier Transform 9.0 "/6
  Counter/1 -> Relational/1
  Up Sample/1 -> "aclken "/1
  Constant4/1 -> Up Sample/1
  "aclken "/1 -> "Fast Fourier Transform 9.0 "/8
  Up Sample1/1 -> s_axis_data_tvalid1/1
  Constant5/1 -> Up Sample1/1
  Gateway Out8/1 -> Scope4/3
  Gateway Out9/1 -> Scope4/4
  Gateway Out1/1 -> Scope4/2
  FIFO/2 -> Gateway Out1/1
  FIFO/3 -> Gateway Out8/1
  FIFO/4 -> Gateway Out9/1
  Gateway Out15/1 -> Scope5/4
  Gateway Out16/1 -> Scope5/5
  Gateway Out14/1 -> Scope5/3
  FIFO1/2 -> Gateway Out14/1
  FIFO1/3 -> Gateway Out15/1
  FIFO1/4 -> Gateway Out16/1
  Gateway Out10/1 -> Scope5/2
  Gateway Out11/1 -> Scope4/1
  Gateway Out12/1 -> Scope5/1
  re2/1 -> FIFO1/3
  Gateway Out13/1 -> Scope5/6
  FIFO1/1 -> Delay1/1, Gateway Out10/1
  FIFO/1 -> Delay4/1, Gateway Out11/1
  Reinterpret3/1 -> FIFO1/1, Gateway Out12/1
  Down Sample5/1 -> Gateway Out13/1, FIFO1/2, FIFO/2
  Constant3/1 -> re1/1, re2/1, db_aft_DMT_Im/1, db_aft_DMT_Re/1
  re1/1 -> FIFO/3
  sg_Im/1 -> Delay/1
  sg_Re/1 -> Delay3/1
  Delay1/1 -> Re_out/1
  Delay4/1 -> Im_out/1

== system Basic_DMT/Sysgen_SIPaFFT/Guard_Interval/None ==
  Re_In : Inport
  Im_In : Inport  Port=2
  Delay : xbsIndex_r4/Delay  Commented=through  rst=off  infoeditControl=Selection of Reset will increase slice count due to use of real FFs and instead of SRLs  en=off  latency=8  reg_retiming=off  dbl_ovrd=off  block_type=delay
  Delay1 : xbsIndex_r4/Delay  Commented=through  rst=off  infoeditControl=Selection of Reset will increase slice count due to use of real FFs and instead of SRLs  en=off  latency=8  reg_retiming=off  dbl_ovrd=off  block_type=delay
  Re : Outport
  Im : Outport  Port=2
  wires:
  Im_In/1 -> Delay1/1
  Re_In/1 -> Delay/1
  Delay/1 -> Re/1
  Delay1/1 -> Im/1
